simulink library "LU_TEG"  (R2015a)
settings: Solver=ode45  StartTime=0.0  StopTime=10.0  RelTol=1e-3
undefined symbols (not defined in the file): a, a_hxr, B, b_hxr, C_ap, C_cxr, C_hxr, ca1, ca2, ca3, cb1, cb2, cb3, ct1, ct2, Di_cxr, f, k_gap, l, l_cw, l_hxr, l_TEM, M, M_ap, M_cxr, M_hxr, n, N, Nf_hxr, P, plate_fin_hxr_A, side, T1, T1_T2, T_cint, T_hint, tf_hxr, Tune_er, Tune_tr
(part 1 of 2)
settings Model: Creator=lansong7  LastModifiedBy=lansong7

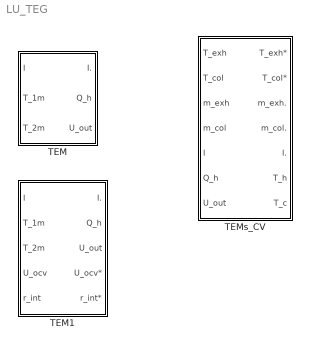
== system LU_TEG ==
  TEM : Subsystem  mask{l=l, l_cw=l_cw, f=f, a=a, n=n, Tune_tr=Tune_tr, Tune_er=Tune_er, ct1=ct1, ct2=ct2}
      mask prompts: l "Length of thermocouples [m]"; l_cw "Cermaic wafer length [m]"; f "Fill factor [-]"; a "Area of a TEM [m2]"; n "Number of thermal couple"; Tune_tr "Tuning for thermal resistance"; Tune_er "Tuning for electrical resistance"; ct1 "Tuning for  contact resistance ct1"; ct2 "Tuning for  contact resistance ct2"
      mask DialogControl ParameterGroupVar_copy Prompt: Geometrical Parameters
      mask DialogControl ParameterGroupVar Prompt: Tuning Parameters
  TEM1 : Subsystem  mask{l=l, l_cw=l_cw, f=f, a=a, n=n, Tune_tr=Tune_tr, Tune_er=Tune_er, ct1=ct1, ct2=ct2, M=M}
      mask prompts: l "Length of thermocouples [m]"; l_cw "Cermaic wafer length [m]"; f "Fill factor [-]"; a "Area of a TEM [m2]"; n "Number of thermal couple"; Tune_tr "Tuning for thermal resistance"; Tune_er "Tuning for electrical resistance"; ct1 "Tuning for  contact resistance ct1"; ct2 "Tuning for  contact resistance ct2"; M "Number of TEMs in a CV"
      mask DialogControl ParameterGroupVar_copy Prompt: Geometrical Parameters
      mask DialogControl ParameterGroupVar Prompt: Tuning Parameters
  TEMs_CV : Subsystem  mask{B=B, a=a, side=side, l_TEM=l_TEM, M=M, M_hxr=M_hxr, M_ap=M_ap, C_hxr=C_hxr, C_ap=C_ap, l_hxr=l_hxr, b_hxr=b_hxr, a_hxr=a_hxr, Nf_hxr=Nf_hxr, tf_hxr=tf_hxr, M_cxr=M_cxr, C_cxr=C_cxr, Di_cxr=Di_cxr, T_hint=T_hint, T_cint=T_cint, ca1=ca1, ca2=ca2, ca3=ca3, cb1=cb1, cb2=cb2, cb3=cb3}
      mask prompts: B "Area of a Control Volume [m2]"; a "Areas of a TEM [m2]"; side "Number of heat exchanger channels"; l_TEM "Length of  a TEM [m]"; M "Number of TEMs in a CV"; M_hxr "Mass of hot side  heat exchanger [kg]"; M_ap "Mass of aluminate plate [kg]"; C_hxr "Heat capacity of of hot side heat exchanger [J/(kg.K)]"; C_ap "Heat capacity of of aluminate plate [J/(kg.K)]"; l_hxr "Length of hot side heat exchanger [m]"; b_hxr "Width of hot side heat exchanger"; a_hxr "Height of hot side heat exchanger"; Nf_hxr "Number of the fins of hot side heat exchanger"; tf_hxr "Fin thickness of hot side heat exchanger"; M_cxr "Mass of cold side  heat exchanger [kg]"; C_cxr "Heat capacity of of cold side heat exchanger [J/(kg.K)]"; Di_cxr "Inner diameter of cold side heat exchanger"; T_hint "Initial temperature of hot side wall"; T_cint "Initial temperature of cold side wall"; ca1 "Tuning constant of hot side transfer coefficient ca1"; ca2 "Tuning constant of hot side transfer coefficient ca2"; ca3 "Tuning constant of hot side transfer coefficient ca3"; cb1 "Tuning constant of cold side transfer coefficient cb1"; cb2 "Tuning constant of cold side transfer coefficient cb2"; cb3 "Tuning constant of cold side transfer coefficient cb3"
      mask DialogControl ParameterGroupVar Prompt: Geometrical Parameters
      mask DialogControl ParameterGroupVar_copy Prompt: Hot side Heat Exchanger Parameters
      mask DialogControl ParameterGroupVar_copy_copy Prompt: Cold side Heat Exchanger Parameters
      mask DialogControl ParameterGroupVar_copy_copy_copy Prompt: Tuning Parameters

== system LU_TEG/TEM ==
  note: 2
  I : Inport  OutDataTypeStr=double  PortDimensions=1  SampleTime=[0,1]
  T_1m : Inport  Port=2  OutDataTypeStr=double  PortDimensions=1  SampleTime=[0,1]
  T_2m : Inport  Port=3  OutDataTypeStr=double  PortDimensions=1  SampleTime=[0,1]
  Spn : Subsystem
  Subsystem4 : Subsystem
  Subsystem5 : Subsystem
  Terminator : Terminator
  Terminator1 : Terminator
  r_int : Subsystem
  I. : Outport  OutDataTypeStr=double  PortDimensions=1  SampleTime=[0,1]
  Q_h : Outport  Port=2  OutDataTypeStr=double  PortDimensions=1  SampleTime=[0,1]
  U_out : Outport  Port=3
  wires:
  Subsystem4/2(Q_h) -> Q_h/1
  I/1 -> Subsystem4/6(I)
  Subsystem4/3(U_out) -> U_out/1
  Spn/1(Spn) -> Subsystem4/7(Spn)
  r_int/1(r_int) -> Subsystem4/8(r_int)
  T_2m/1 -> r_int/2(T_2m), Spn/2(T_2m), Subsystem5/2(T_2m), Subsystem4/2(T_2m)
  Subsystem5/1(Rcw1) -> Subsystem4/3(Rh)
  Subsystem5/3(Rt) -> Subsystem4/5(Rt)
  Subsystem5/2(Rcw2) -> Subsystem4/4(Rc)
  Subsystem4/4(U_ocv) -> Terminator/1
  Subsystem4/1(I.) -> I./1
  Subsystem4/5(r_int.) -> Terminator1/1
  T_1m/1 -> r_int/1(T_1m), Spn/1(T_1m), Subsystem5/1(T_1m), Subsystem4/1(T_1m)

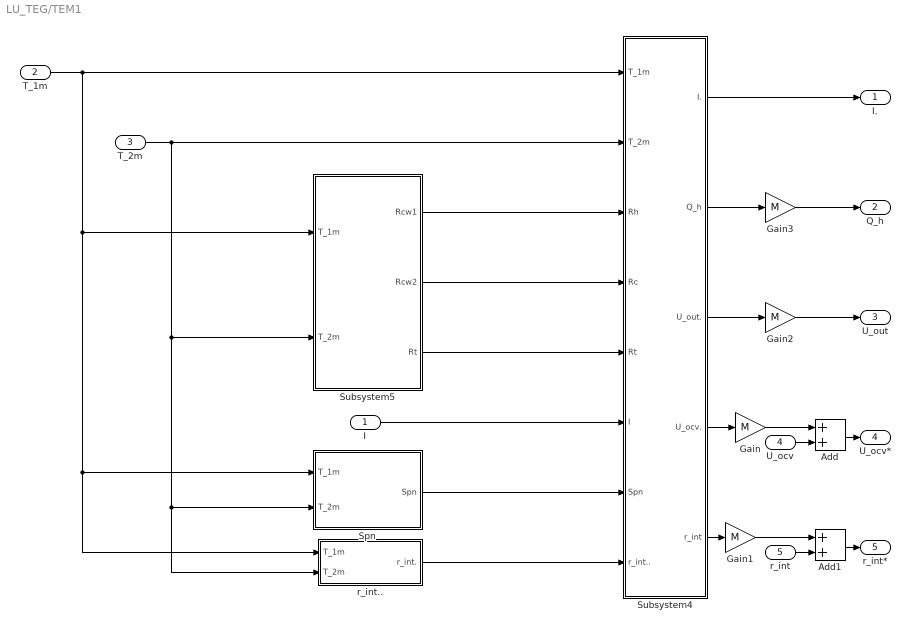
== system LU_TEG/TEM1 ==
  I : Inport  OutDataTypeStr=double  PortDimensions=1  SampleTime=[0,1]
  T_1m : Inport  Port=2  OutDataTypeStr=double  PortDimensions=1  SampleTime=[0,1]
  T_2m : Inport  Port=3  OutDataTypeStr=double  PortDimensions=1  SampleTime=[0,1]
  U_ocv : Inport  Port=4  OutDataTypeStr=double  PortDimensions=1  SampleTime=[0,1]
  r_int : Inport  Port=5  OutDataTypeStr=double  PortDimensions=1  SampleTime=[0,1]
  Add : Sum
  Add1 : Sum
  Gain{,1..3} (4 alike) : Gain  Gain=M
  Spn : Subsystem
  Subsystem4 : Subsystem
  Subsystem5 : Subsystem
  r_int.. : Subsystem
  I. : Outport  OutDataTypeStr=double  PortDimensions=1  SampleTime=[0,1]
  Q_h : Outport  Port=2  OutDataTypeStr=double  PortDimensions=1  SampleTime=[0,1]
  U_out : Outport  Port=3
  U_ocv* : Outport  Port=4
  "r_int* " : Outport  Port=5
  wires:
  T_1m/1 -> Subsystem4/1(T_1m), Subsystem5/1(T_1m), Spn/1(T_1m), r_int../1(T_1m)
  Subsystem4/1(I.) -> I./1
  Subsystem5/2(Rcw2) -> Subsystem4/4(Rc)
  Subsystem5/3(Rt) -> Subsystem4/5(Rt)
  Subsystem5/1(Rcw1) -> Subsystem4/3(Rh)
  T_2m/1 -> Subsystem4/2(T_2m), Subsystem5/2(T_2m), Spn/2(T_2m), r_int../2(T_2m)
  r_int../1(r_int.) -> Subsystem4/8(r_int..)
  Spn/1(Spn) -> Subsystem4/7(Spn)
  Subsystem4/3(U_out.) -> Gain2/1
  I/1 -> Subsystem4/6(I)
  Subsystem4/2(Q_h) -> Gain3/1
  Subsystem4/4(U_ocv.) -> Gain/1
  U_ocv/1 -> Add/2
  Subsystem4/5(r_int) -> Gain1/1
  r_int/1 -> Add1/2
  Gain2/1 -> U_out/1
  Gain3/1 -> Q_h/1
  Gain/1 -> Add/1
  Add/1 -> U_ocv*/1
  Gain1/1 -> Add1/1
  Add1/1 -> "r_int* "/1

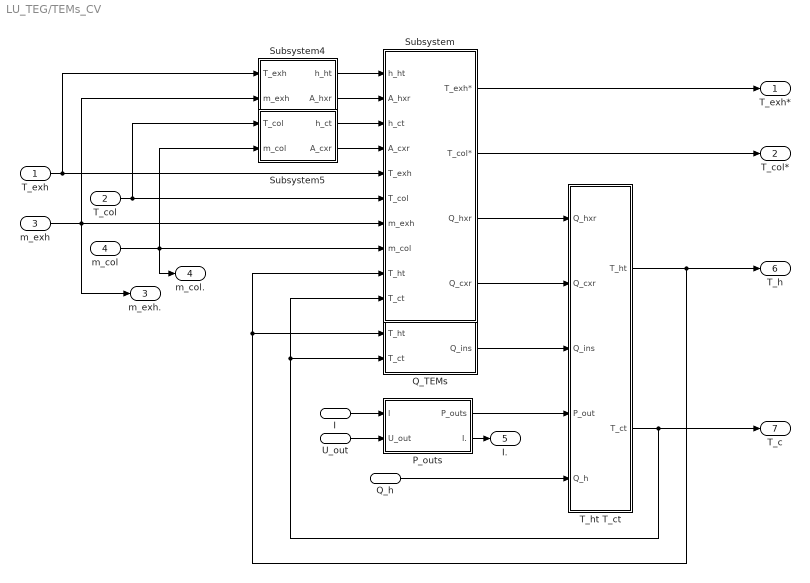
== system LU_TEG/TEMs_CV ==
  T_exh : Inport
  T_col : Inport  Port=2
  m_exh : Inport  Port=3
  m_col : Inport  Port=4
  I : Inport  Port=5
  Q_h : Inport  Port=6
  U_out : Inport  Port=7
  P_outs : Subsystem
  Q_TEMs : Subsystem
  Subsystem : Subsystem
  Subsystem4 : Subsystem
  Subsystem5 : Subsystem
  T_ht T_ct : Subsystem
  T_exh* : Outport
  T_col* : Outport  Port=2
  m_exh. : Outport  Port=3
  m_col. : Outport  Port=4
  I. : Outport  Port=5
  T_h : Outport  Port=6
  T_c : Outport  Port=7
  wires:
  T_exh/1 -> Subsystem4/1(T_exh), Subsystem/5(T_exh)
  T_col/1 -> Subsystem5/1(T_col), Subsystem/6(T_col)
  m_exh/1 -> Subsystem4/2(m_exh), Subsystem/7(m_exh), m_exh./1
  m_col/1 -> m_col./1, Subsystem5/2(m_col), Subsystem/8(m_col)
  Subsystem/1(T_exh*) -> T_exh*/1
  Subsystem/2(T_col*) -> T_col*/1
  Q_TEMs/1(Q_ins) -> T_ht T_ct/3(Q_ins)
  Subsystem/3(Q_hxr) -> T_ht T_ct/1(Q_hxr)
  Subsystem/4(Q_cxr) -> T_ht T_ct/2(Q_cxr)
  I/1 -> P_outs/1(I)
  U_out/1 -> P_outs/2(U_out)
  P_outs/1(P_outs) -> T_ht T_ct/4(P_out)
  P_outs/2(I.) -> I./1
  T_ht T_ct/2(T_ct) -> Subsystem/10(T_ct), Q_TEMs/2(T_ct), T_c/1
  T_ht T_ct/1(T_ht) -> Subsystem/9(T_ht), Q_TEMs/1(T_ht), T_h/1
  Subsystem4/2(A_hxr) -> Subsystem/2(A_hxr)
  Subsystem5/1(h_ct) -> Subsystem/3(h_ct)
  Subsystem5/2(A_cxr) -> Subsystem/4(A_cxr)
  Subsystem4/1(h_ht) -> Subsystem/1(h_ht)
  Q_h/1 -> T_ht T_ct/5(Q_h)

== system LU_TEG/TEM/Spn ==
  T_1m : Inport
  T_2m : Inport  Port=2
  Add : Sum  Inputs=+-
  Add2 : Sum
  Constant2 : Constant  Value=n
  Gain : Gain  Gain=0.5
  Product : Product
  sn : Lookup_n-D  NumberOfTableDimensions=1  BreakpointsForDimension1=N(:,1)  Table=N(:,2)  InterpMethod=Cubic spline  ExtrapMethod=Cubic spline  InternalRulePriority=Speed  RndMeth=Simplest  InputSameDT=on
  sp : Lookup_n-D  NumberOfTableDimensions=1  BreakpointsForDimension1=P(:,1)  Table=P(:,2)  InterpMethod=Cubic spline  ExtrapMethod=Cubic spline  InternalRulePriority=Speed  RndMeth=Simplest  InputSameDT=on
  Spn : Outport
  wires:
  sn/1 -> Add/2
  sp/1 -> Add/1
  Constant2/1 -> Product/1
  Product/1 -> Spn/1
  Add2/1 -> Gain/1
  Gain/1 -> sp/1, sn/1
  T_1m/1 -> Add2/1
  T_2m/1 -> Add2/2
  Add/1 -> Product/2

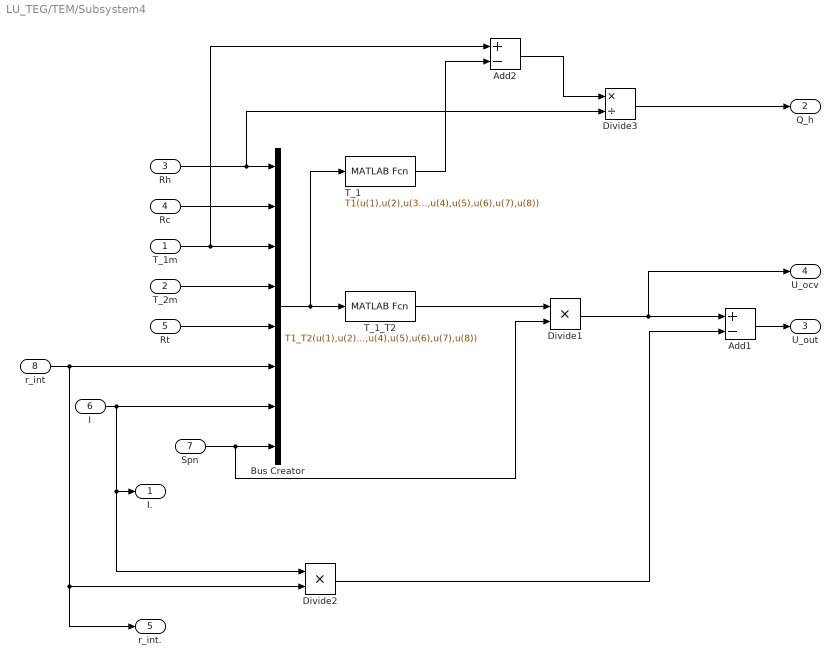
== system LU_TEG/TEM/Subsystem4 ==
  T_1m : Inport
  T_2m : Inport  Port=2
  Rh : Inport  Port=3
  Rc : Inport  Port=4
  Rt : Inport  Port=5
  I : Inport  Port=6
  Spn : Inport  Port=7
  r_int : Inport  Port=8
  Add1 : Sum  Inputs=+-
  Add2 : Sum  Inputs=+-
  Bus Creator : BusCreator  Inputs=8
  Divide1 : Product  Inputs=**
  Divide2 : Product  Inputs=**
  Divide3 : Product  Inputs=*/
  T_1 : MATLABFcn  MATLABFcn=T1(u(1),u(2),u(3),u(4),u(5),u(6),u(7),u(8))  OutputSignalType=real
  T_1_T2 : MATLABFcn  MATLABFcn=T1_T2(u(1),u(2),u(3),u(4),u(5),u(6),u(7),u(8))  OutputSignalType=real
  I. : Outport  OutDataTypeStr=double  PortDimensions=1  SampleTime=[0,1]
  Q_h : Outport  Port=2  OutDataTypeStr=double  PortDimensions=1  SampleTime=[0,1]
  U_out : Outport  Port=3
  U_ocv : Outport  Port=4
  r_int. : Outport  Port=5  OutDataTypeStr=double  PortDimensions=1  SampleTime=[0,1]
  wires:
  r_int/1 -> Bus Creator/6, Divide2/2, r_int./1
  Rh/1 -> Divide3/2, Bus Creator/1
  Rc/1 -> Bus Creator/2
  Rt/1 -> Bus Creator/5
  T_2m/1 -> Bus Creator/4
  T_1m/1 -> Add2/1, Bus Creator/3
  I/1 -> Bus Creator/7, Divide2/1, I./1
  Divide2/1 -> Add1/2
  Add1/1 -> U_out/1
  Spn/1 -> Bus Creator/8, Divide1/2
  Divide1/1 -> U_ocv/1, Add1/1
  T_1_T2/1 -> Divide1/1
  Bus Creator/1 -> T_1/1, T_1_T2/1
  T_1/1 -> Add2/2
  Divide3/1 -> Q_h/1
  Add2/1 -> Divide3/1

== system LU_TEG/TEM/Subsystem5 ==
  T_1m : Inport
  T_2m : Inport  Port=2
  R_cw : Subsystem
  Rt. : Subsystem
  Rcw1 : Outport
  Rcw2 : Outport  Port=2
  Rt : Outport  Port=3
  wires:
  R_cw/1(Rcw1) -> Rcw1/1
  Rt./1(Rt) -> Rt/1
  R_cw/2(Rcw2) -> Rcw2/1
  T_2m/1 -> R_cw/2(T_2m), Rt./2(T_2m)
  T_1m/1 -> R_cw/1(T_1m), Rt./1(T_1m)

== system LU_TEG/TEM/r_int ==
  T_1m : Inport
  T_2m : Inport  Port=2
  Add2 : Sum
  Add4 : Sum
  Constant12 : Constant  Value=0.5*a*f/n
  Constant13 : Constant  Value=0.5*a*f/n
  Constant14 : Constant  Value=l
  Constant16 : Constant  Value=l
  Constant18 : Constant  Value=n
  Constant4 : Constant  Value=n
  Gain : Gain  Gain=Tune_er
  Gain1 : Gain  Gain=0.5
  Product3 : Product  Inputs=***/
  Product4 : Product  Inputs=***/
  rhon : Lookup_n-D  NumberOfTableDimensions=1  BreakpointsForDimension1=N(:,1)  Table=N(:,3)  InterpMethod=Cubic spline  ExtrapMethod=Cubic spline  InternalRulePriority=Speed  RndMeth=Simplest  InputSameDT=on
  rhop : Lookup_n-D  NumberOfTableDimensions=1  BreakpointsForDimension1=P(:,1)  Table=P(:,3)  InterpMethod=Cubic spline  ExtrapMethod=Cubic spline  InternalRulePriority=Speed  RndMeth=Simplest  InputSameDT=on
  r_int : Outport
  wires:
  Constant18/1 -> Product4/1
  Constant14/1 -> Product3/2
  rhop/1 -> Product3/3
  Constant12/1 -> Product3/4
  rhon/1 -> Product4/3
  Constant13/1 -> Product4/4
  Constant4/1 -> Product3/1
  Constant16/1 -> Product4/2
  Product3/1 -> Add2/1
  Product4/1 -> Add2/2
  T_1m/1 -> Add4/1
  T_2m/1 -> Add4/2
  Add4/1 -> Gain1/1
  Add2/1 -> Gain/1
  Gain1/1 -> rhon/1, rhop/1
  Gain/1 -> r_int/1

== system LU_TEG/TEM1/Spn ==
  T_1m : Inport
  T_2m : Inport  Port=2
  Add : Sum  Inputs=+-
  Add2 : Sum
  Constant2 : Constant  Value=n
  Gain : Gain  Gain=0.5
  Product : Product
  sn : Lookup_n-D  NumberOfTableDimensions=1  BreakpointsForDimension1=N(:,1)  Table=N(:,2)  InterpMethod=Cubic spline  ExtrapMethod=Cubic spline  InternalRulePriority=Speed  RndMeth=Simplest  InputSameDT=on
  sp : Lookup_n-D  NumberOfTableDimensions=1  BreakpointsForDimension1=P(:,1)  Table=P(:,2)  InterpMethod=Cubic spline  ExtrapMethod=Cubic spline  InternalRulePriority=Speed  RndMeth=Simplest  InputSameDT=on
  Spn : Outport
  wires:
  Add/1 -> Product/2
  T_2m/1 -> Add2/2
  T_1m/1 -> Add2/1
  Gain/1 -> sn/1, sp/1
  Add2/1 -> Gain/1
  Product/1 -> Spn/1
  Constant2/1 -> Product/1
  sp/1 -> Add/1
  sn/1 -> Add/2

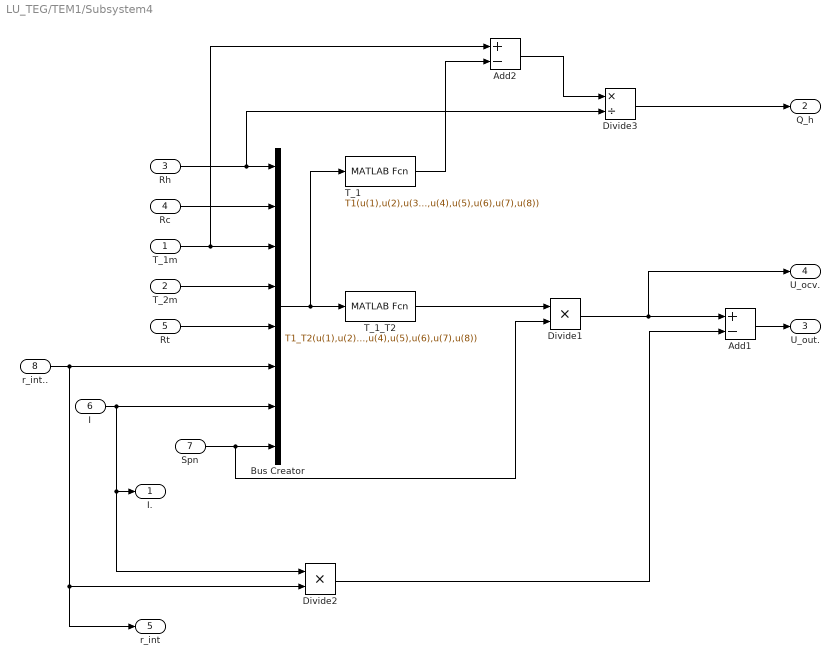
== system LU_TEG/TEM1/Subsystem4 ==
  T_1m : Inport
  T_2m : Inport  Port=2
  Rh : Inport  Port=3
  Rc : Inport  Port=4
  Rt : Inport  Port=5
  I : Inport  Port=6
  Spn : Inport  Port=7
  r_int.. : Inport  Port=8
  Add1 : Sum  Inputs=+-
  Add2 : Sum  Inputs=+-
  Bus Creator : BusCreator  Inputs=8
  Divide1 : Product  Inputs=**
  Divide2 : Product  Inputs=**
  Divide3 : Product  Inputs=*/
  T_1 : MATLABFcn  MATLABFcn=T1(u(1),u(2),u(3),u(4),u(5),u(6),u(7),u(8))  OutputSignalType=real
  T_1_T2 : MATLABFcn  MATLABFcn=T1_T2(u(1),u(2),u(3),u(4),u(5),u(6),u(7),u(8))  OutputSignalType=real
  I. : Outport  OutDataTypeStr=double  PortDimensions=1  SampleTime=[0,1]
  Q_h : Outport  Port=2  OutDataTypeStr=double  PortDimensions=1  SampleTime=[0,1]
  U_out. : Outport  Port=3
  U_ocv. : Outport  Port=4
  r_int : Outport  Port=5  OutDataTypeStr=double  PortDimensions=1  SampleTime=[0,1]
  wires:
  Add2/1 -> Divide3/1
  Divide3/1 -> Q_h/1
  T_1/1 -> Add2/2
  Bus Creator/1 -> T_1_T2/1, T_1/1
  T_1_T2/1 -> Divide1/1
  Divide1/1 -> Add1/1, U_ocv./1
  Spn/1 -> Divide1/2, Bus Creator/8
  Add1/1 -> U_out./1
  Divide2/1 -> Add1/2
  I/1 -> I./1, Divide2/1, Bus Creator/7
  T_1m/1 -> Bus Creator/3, Add2/1
  T_2m/1 -> Bus Creator/4
  Rt/1 -> Bus Creator/5
  Rc/1 -> Bus Creator/2
  Rh/1 -> Bus Creator/1, Divide3/2
  r_int../1 -> r_int/1, Divide2/2, Bus Creator/6

== system LU_TEG/TEM1/Subsystem5 ==
  T_1m : Inport
  T_2m : Inport  Port=2
  R_cw : Subsystem
  Rt. : Subsystem
  Rcw1 : Outport
  Rcw2 : Outport  Port=2
  Rt : Outport  Port=3
  wires:
  T_1m/1 -> Rt./1(T_1m), R_cw/1(T_1m)
  T_2m/1 -> Rt./2(T_2m), R_cw/2(T_2m)
  R_cw/2(Rcw2) -> Rcw2/1
  Rt./1(Rt) -> Rt/1
  R_cw/1(Rcw1) -> Rcw1/1

== system LU_TEG/TEM1/r_int.. ==
  T_1m : Inport
  T_2m : Inport  Port=2
  Add2 : Sum
  Add4 : Sum
  Constant12 : Constant  Value=0.5*a*f/n
  Constant13 : Constant  Value=0.5*a*f/n
  Constant14 : Constant  Value=l
  Constant16 : Constant  Value=l
  Constant18 : Constant  Value=n
  Constant4 : Constant  Value=n
  Gain : Gain  Gain=Tune_er
  Gain1 : Gain  Gain=0.5
  Product3 : Product  Inputs=***/
  Product4 : Product  Inputs=***/
  rhon : Lookup_n-D  NumberOfTableDimensions=1  BreakpointsForDimension1=N(:,1)  Table=N(:,3)  InterpMethod=Cubic spline  ExtrapMethod=Cubic spline  InternalRulePriority=Speed  RndMeth=Simplest  InputSameDT=on
  rhop : Lookup_n-D  NumberOfTableDimensions=1  BreakpointsForDimension1=P(:,1)  Table=P(:,3)  InterpMethod=Cubic spline  ExtrapMethod=Cubic spline  InternalRulePriority=Speed  RndMeth=Simplest  InputSameDT=on
  r_int. : Outport
  wires:
  Gain/1 -> r_int./1
  Gain1/1 -> rhop/1, rhon/1
  Add2/1 -> Gain/1
  Add4/1 -> Gain1/1
  T_2m/1 -> Add4/2
  T_1m/1 -> Add4/1
  Product4/1 -> Add2/2
  Product3/1 -> Add2/1
  Constant16/1 -> Product4/2
  Constant4/1 -> Product3/1
  Constant13/1 -> Product4/4
  rhon/1 -> Product4/3
  Constant12/1 -> Product3/4
  rhop/1 -> Product3/3
  Constant14/1 -> Product3/2
  Constant18/1 -> Product4/1

== system LU_TEG/TEMs_CV/P_outs ==
  I : Inport
  U_out : Inport  Port=2
  Divide : Product  Inputs=**
  P_outs : Outport
  I. : Outport  Port=2
  wires:
  Divide/1 -> P_outs/1
  I/1 -> I./1, Divide/2
  U_out/1 -> Divide/1

== system LU_TEG/TEMs_CV/Q_TEMs ==
  T_ht : Inport
  T_ct : Inport  Port=2
  Q_TEMs. : Subsystem
  Q_ins : Outport
  wires:
  T_ht/1 -> Q_TEMs./1(T_ht)
  T_ct/1 -> Q_TEMs./2(T_ct)
  Q_TEMs./1(Q_ins) -> Q_ins/1

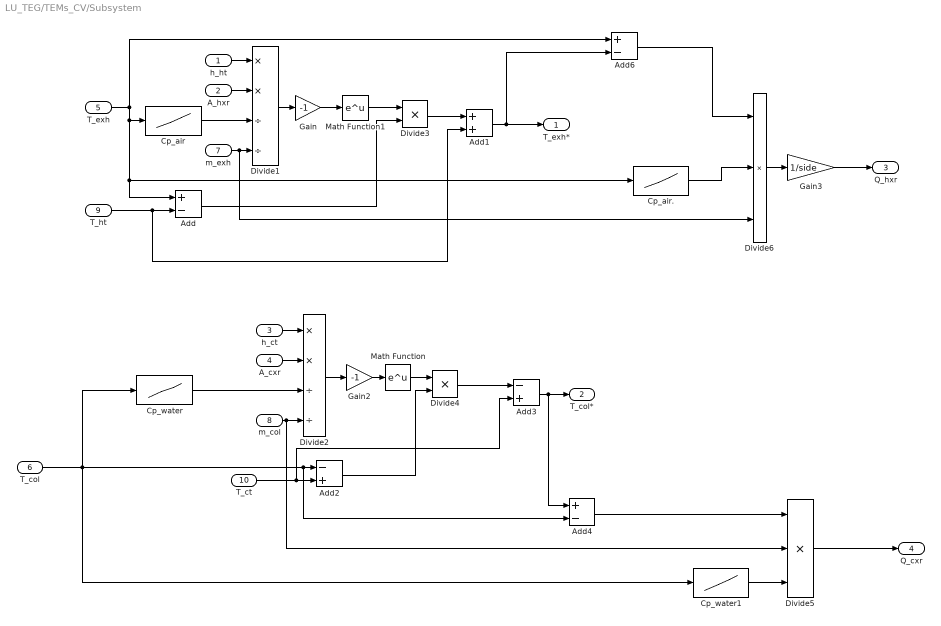
== system LU_TEG/TEMs_CV/Subsystem ==
  h_ht : Inport
  A_hxr : Inport  Port=2
  h_ct : Inport  Port=3
  A_cxr : Inport  Port=4
  T_exh : Inport  Port=5
  T_col : Inport  Port=6
  m_exh : Inport  Port=7
  m_col : Inport  Port=8
  T_ht : Inport  Port=9
  T_ct : Inport  Port=10
  Add : Sum  Inputs=+-
  Add1 : Sum
  Add2 : Sum  Inputs=-+
  Add3 : Sum  Inputs=-+
  Add4 : Sum  Inputs=+-
  Add6 : Sum  Inputs=+-
  Cp_air : Lookup_n-D  NumberOfTableDimensions=1  BreakpointsForDimension1=|  Table=|  InterpMethod=Cubic spline  ExtrapMethod=Cubic spline  RndMeth=Simplest  InputSameDT=on
      BreakpointsForDimension1=|
      | [293
      | 313
      | 333
      | 353
      | 373
      | 393
      | 413
      | 433
      | 453
      | 473
      | 493
      | 513
      | 533
      | 553
      | 573
      | 593
      | 613
      | 633
      | 653
      | 673
      | 693
      | 713
      | 733
      | 753
      | 773
      | 793
      | 813
      | 833
      | 853
      | 873
      | 900
      | 920
      | 940
      | 960
      | 980
      | 1000
      | 1020
      | 1040
      | 1060
      | 1080
      | 1100
      | 1120
      | 1140
      | 1160
      | 1180
      | 1200
      | 1220
      | 1240
      | 1260
      | 1280
      | 1300
      | 1320
      | 1340
      | 1360
      | 1380
      | 1400
      | 1420
      | 1440
      | 1460
      | 1480]
      Table=|
      | [1007
      | 1008
      | 1008
      | 1009
      | 1011
      | 1013
      | 1016
      | 1019
      | 1023
      | 1026
      | 1029
      | 1033
      | 1036
      | 1041
      | 1046
      | 1050
      | 1055
      | 1059
      | 1064
      | 1069
      | 1073
      | 1078
      | 1082
      | 1088
      | 1093
      | 1097
      | 1102
      | 1106
      | 1111
      | 1115
      | 1121
      | 1125
      | 1129
      | 1133
      | 1137
      | 1141
      | 1145
      | 1148
      | 1152
      | 1155
      | 1159
      | 1162
      | 1165
      | 1168
      | 1171
      | 1174
      | 1177
      | 1180
      | 1183
      | 1185
      | 1188
      | 1191
      | 1193
      | 1196
      | 1198
      | 1200
      | 1202
      | 1205
      | 1207
      | 1209
      | ]
  Cp_air. : Lookup_n-D  NumberOfTableDimensions=1  BreakpointsForDimension1=|  Table=|  InterpMethod=Cubic spline  ExtrapMethod=Cubic spline  RndMeth=Simplest  InputSameDT=on
      BreakpointsForDimension1=|
      | [293
      | 313
      | 333
      | 353
      | 373
      | 393
      | 413
      | 433
      | 453
      | 473
      | 493
      | 513
      | 533
      | 553
      | 573
      | 593
      | 613
      | 633
      | 653
      | 673
      | 693
      | 713
      | 733
      | 753
      | 773
      | 793
      | 813
      | 833
      | 853
      | 873
      | 900
      | 920
      | 940
      | 960
      | 980
      | 1000
      | 1020
      | 1040
      | 1060
      | 1080
      | 1100
      | 1120
      | 1140
      | 1160
      | 1180
      | 1200
      | 1220
      | 1240
      | 1260
      | 1280
      | 1300
      | 1320
      | 1340
      | 1360
      | 1380
      | 1400
      | 1420
      | 1440
      | 1460
      | 1480]
      Table=|
      | [1007
      | 1008
      | 1008
      | 1009
      | 1011
      | 1013
      | 1016
      | 1019
      | 1023
      | 1026
      | 1029
      | 1033
      | 1036
      | 1041
      | 1046
      | 1050
      | 1055
      | 1059
      | 1064
      | 1069
      | 1073
      | 1078
      | 1082
      | 1088
      | 1093
      | 1097
      | 1102
      | 1106
      | 1111
      | 1115
      | 1121
      | 1125
      | 1129
      | 1133
      | 1137
      | 1141
      | 1145
      | 1148
      | 1152
      | 1155
      | 1159
      | 1162
      | 1165
      | 1168
      | 1171
      | 1174
      | 1177
      | 1180
      | 1183
      | 1185
      | 1188
      | 1191
      | 1193
      | 1196
      | 1198
      | 1200
      | 1202
      | 1205
      | 1207
      | 1209
      | ]
  Cp_water : Lookup_n-D  NumberOfTableDimensions=1  BreakpointsForDimension1=|  Table=|  InterpMethod=Cubic spline  ExtrapMethod=Cubic spline  RndMeth=Simplest  InputSameDT=on
      BreakpointsForDimension1=|
      | [273
      | 274
      | 275
      | 276
      | 277
      | 278
      | 279
      | 280
      | 281
      | 282
      | 283
      | 284
      | 285
      | 286
      | 287
      | 288
      | 289
      | 290
      | 291
      | 292
      | 293
      | 294
      | 295
      | 296
      | 297
      | 298
      | 299
      | 300
      | 301
      | 302
      | 303
      | 304
      | 305
      | 306
      | 307
      | 308
      | 309
      | 310
      | 311
      | 312
      | 313
      | 314
      | 315
      | 316
      | 317
      | 318
      | 319
      | 320
      | 321
      | 322
      | 323
      | 324
      | 325
      | 326
      | 327
      | 328
      | 329
      | 330
      | 331
      | 332
      | 333
      | 334
      | 335
      | 336
      | 337
      | 338
      | 339
      | 340
      | 341
      | 342
      | 343
      | 344
      | 345
      | 346
      | 347
      | 348
      | 349
      | 350
      | 351
      | 352
      | 353
      | 354
      | 355
      | 356
      | 357
      | 358
      | 359
      | 360
      | 361
      | 362
      | 363
      | 364
      | 365
      | 366
      | 367
      | 368
      | 369
      | 370
      | 371
      | 372
      | 373]
      Table=|
      | [4217
      | 4213
      | 4210
      | 4207
      | 4205
      | 4202
      | 4200
      | 4198
      | 4196
      | 4194
      | 4192
      | 4191
      | 4189
      | 4188
      | 4187
      | 4186
      | 4185
      | 4184
      | 4183
      | 4182
      | 4182
      | 4181
      | 4181
      | 4180
      | 4180
      | 4180
      | 4179
      | 4179
      | 4179
      | 4179
      | 4178
      | 4178
      | 4178
      | 4178
      | 4178
      | 4178
      | 4178
      | 4178
      | 4178
      | 4179
      | 4179
      | 4179
      | 4179
      | 4179
      | 4179
      | 4180
      | 4180
      | 4180
      | 4180
      | 4181
      | 4181
      | 4181
      | 4182
      | 4182
      | 4182
      | 4183
      | 4183
      | 4183
      | 4184
      | 4184
      | 4185
      | 4185
      | 4186
      | 4186
      | 4187
      | 4187
      | 4188
      | 4188
      | 4189
      | 4189
      | 4190
      | 4190
      | 4191
      | 4192
      | 4192
      | 4193
      | 4194
      | 4194
      | 4195
      | 4196
      | 4196
      | 4197
      | 4198
      | 4199
      | 4200
      | 4200
      | 4201
      | 4202
      | 4203
      | 4204
      | 4205
      | 4206
      | 4207
      | 4208
      | 4209
      | 4210
      | 4211
      | 4212
      | 4213
      | 4214
      | 4216]
  Cp_water1 : Lookup_n-D  NumberOfTableDimensions=1  BreakpointsForDimension1=|  Table=|  InterpMethod=Cubic spline  ExtrapMethod=Cubic spline  RndMeth=Simplest  InputSameDT=on
      BreakpointsForDimension1=|
      | [273
      | 274
      | 275
      | 276
      | 277
      | 278
      | 279
      | 280
      | 281
      | 282
      | 283
      | 284
      | 285
      | 286
      | 287
      | 288
      | 289
      | 290
      | 291
      | 292
      | 293
      | 294
      | 295
      | 296
      | 297
      | 298
      | 299
      | 300
      | 301
      | 302
      | 303
      | 304
      | 305
      | 306
      | 307
      | 308
      | 309
      | 310
      | 311
      | 312
      | 313
      | 314
      | 315
      | 316
      | 317
      | 318
      | 319
      | 320
      | 321
      | 322
      | 323
      | 324
      | 325
      | 326
      | 327
      | 328
      | 329
      | 330
      | 331
      | 332
      | 333
      | 334
      | 335
      | 336
      | 337
      | 338
      | 339
      | 340
      | 341
      | 342
      | 343
      | 344
      | 345
      | 346
      | 347
      | 348
      | 349
      | 350
      | 351
      | 352
      | 353
      | 354
      | 355
      | 356
      | 357
      | 358
      | 359
      | 360
      | 361
      | 362
      | 363
      | 364
      | 365
      | 366
      | 367
      | 368
      | 369
      | 370
      | 371
      | 372
      | 373]
      Table=|
      | [4217
      | 4213
      | 4210
      | 4207
      | 4205
      | 4202
      | 4200
      | 4198
      | 4196
      | 4194
      | 4192
      | 4191
      | 4189
      | 4188
      | 4187
      | 4186
      | 4185
      | 4184
      | 4183
      | 4182
      | 4182
      | 4181
      | 4181
      | 4180
      | 4180
      | 4180
      | 4179
      | 4179
      | 4179
      | 4179
      | 4178
      | 4178
      | 4178
      | 4178
      | 4178
      | 4178
      | 4178
      | 4178
      | 4178
      | 4179
      | 4179
      | 4179
      | 4179
      | 4179
      | 4179
      | 4180
      | 4180
      | 4180
      | 4180
      | 4181
      | 4181
      | 4181
      | 4182
      | 4182
      | 4182
      | 4183
      | 4183
      | 4183
      | 4184
      | 4184
      | 4185
      | 4185
      | 4186
      | 4186
      | 4187
      | 4187
      | 4188
      | 4188
      | 4189
      | 4189
      | 4190
      | 4190
      | 4191
      | 4192
      | 4192
      | 4193
      | 4194
      | 4194
      | 4195
      | 4196
      | 4196
      | 4197
      | 4198
      | 4199
      | 4200
      | 4200
      | 4201
      | 4202
      | 4203
      | 4204
      | 4205
      | 4206
      | 4207
      | 4208
      | 4209
      | 4210
      | 4211
      | 4212
      | 4213
      | 4214
      | 4216]
  Divide1 : Product  Inputs=**//
  Divide2 : Product  Inputs=**//
  Divide3 : Product  Inputs=**
  Divide4 : Product  Inputs=**
  Divide5 : Product  Inputs=***
  Divide6 : Product  Inputs=***
  Gain : Gain  Gain=-1
  Gain2 : Gain  Gain=-1
  Gain3 : Gain  Gain=1/side
  Math Function : Math  SaturateOnIntegerOverflow=on
  Math Function1 : Math  SaturateOnIntegerOverflow=on
  T_exh* : Outport
  T_col* : Outport  Port=2
  Q_hxr : Outport  Port=3
  Q_cxr : Outport  Port=4
  wires:
  Gain/1 -> Math Function1/1
  A_hxr/1 -> Divide1/2
  Add/1 -> Divide3/2
  m_col/1 -> Divide5/2, Divide2/4
  Divide4/1 -> Add3/1
  T_ht/1 -> Add1/2, Add/2
  Math Function1/1 -> Divide3/1
  Divide3/1 -> Add1/1
  Add1/1 -> Add6/2, T_exh*/1
  Add2/1 -> Divide4/2
  h_ht/1 -> Divide1/1
  Divide2/1 -> Gain2/1
  Cp_air/1 -> Divide1/3
  Add3/1 -> Add4/1, T_col*/1
  Cp_water/1 -> Divide2/3
  h_ct/1 -> Divide2/1
  A_cxr/1 -> Divide2/2
  Divide1/1 -> Gain/1
  m_exh/1 -> Divide6/3, Divide1/4
  Math Function/1 -> Divide4/1
  T_ct/1 -> Add3/2, Add2/2
  Gain2/1 -> Math Function/1
  Cp_water1/1 -> Divide5/3
  Add4/1 -> Divide5/1
  T_exh/1 -> Cp_air./1, Add/1, Cp_air/1, Add6/1
  Cp_air./1 -> Divide6/2
  Add6/1 -> Divide6/1
  Divide6/1 -> Gain3/1
  Gain3/1 -> Q_hxr/1
  Divide5/1 -> Q_cxr/1
  T_col/1 -> Cp_water1/1, Add4/2, Add2/1, Cp_water/1

== system LU_TEG/TEMs_CV/Subsystem4 ==
  T_exh : Inport
  m_exh : Inport  Port=2
  A. : MATLABFcn  MATLABFcn=plate_fin_hxr_A(u(1),u(2),u(3),u(4),u(5),u(6),u(7))
  Bus Creator1 : BusCreator  Inputs=7
  Constant2 : Constant  Value=l_hxr
  Constant3 : Constant  Value=b_hxr
  Constant4 : Constant  Value=a_hxr
  Constant5 : Constant  Value=Nf_hxr
  Constant6 : Constant  Value=tf_hxr
  Subsystem3 : Subsystem
  k_stainless : Lookup_n-D  NumberOfTableDimensions=1  BreakpointsForDimension1=|  Table=|  InterpMethod=Cubic spline  ExtrapMethod=Cubic spline  RndMeth=Simplest  InputSameDT=on
      BreakpointsForDimension1=|
      | [100.0
      | 200.0
      | 300.0
      | 400.0
      | 600.0
      | 800.0
      | 1000.0
      | 1200.0
      | 1500.0
      | ]
      Table=|
      | [9.2
      | 12.6
      | 14.9
      | 16.6
      | 19.8
      | 22.6
      | 25.4
      | 28.0
      | 31.7
      | ]
  h_ht : Outport
  A_hxr : Outport  Port=2
  wires:
  Constant6/1 -> Bus Creator1/5
  Constant2/1 -> Bus Creator1/1
  k_stainless/1 -> Bus Creator1/6
  Constant5/1 -> Bus Creator1/4
  m_exh/1 -> Subsystem3/2(m_exh)
  Constant4/1 -> Bus Creator1/3
  Bus Creator1/1 -> A./1
  Constant3/1 -> Bus Creator1/2
  A./1 -> A_hxr/1
  Subsystem3/1(h_exh) -> h_ht/1, Bus Creator1/7
  T_exh/1 -> k_stainless/1, Subsystem3/1(T_exh)

== system LU_TEG/TEMs_CV/Subsystem5 ==
  T_col : Inport
  m_col : Inport  Port=2
  Constant : Constant  Value=l_hxr*b_hxr
  Subsystem3 : Subsystem
  h_ct : Outport
  A_cxr : Outport  Port=2
  wires:
  m_col/1 -> Subsystem3/2(m_col)
  Constant/1 -> A_cxr/1
  Subsystem3/1(h_col) -> h_ct/1
  T_col/1 -> Subsystem3/1(T_col)

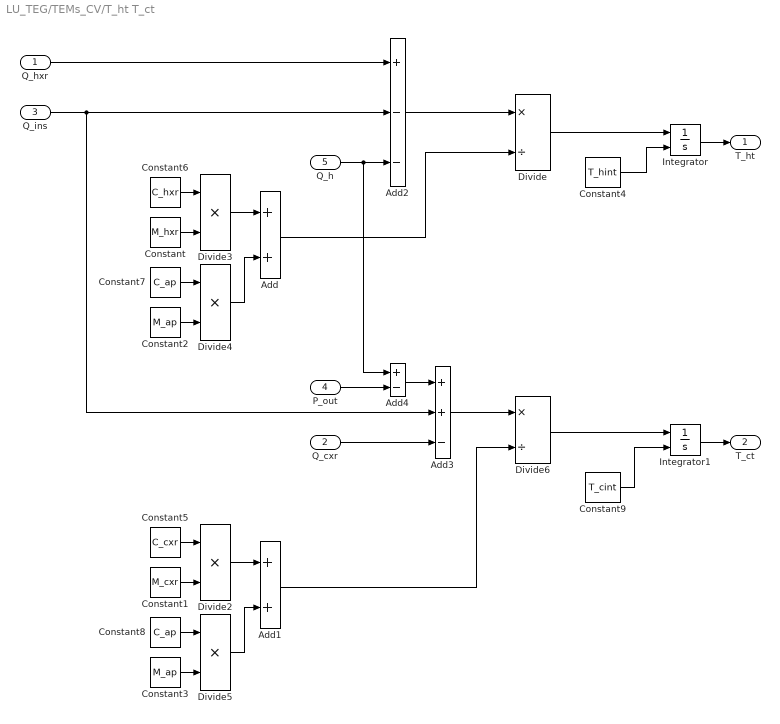
== system LU_TEG/TEMs_CV/T_ht T_ct ==
  Q_hxr : Inport
  Q_cxr : Inport  Port=2
  Q_ins : Inport  Port=3
  P_out : Inport  Port=4
  Q_h : Inport  Port=5
  Add : Sum
  Add1 : Sum
  Add2 : Sum  Inputs=+--
  Add3 : Sum  Inputs=++-
  Add4 : Sum  Inputs=+-
  Constant : Constant  Value=M_hxr
  Constant1 : Constant  Value=M_cxr
  Constant2 : Constant  Value=M_ap
  Constant3 : Constant  Value=M_ap
  Constant4 : Constant  Value=T_hint
  Constant5 : Constant  Value=C_cxr
  Constant6 : Constant  Value=C_hxr
  Constant7 : Constant  Value=C_ap
  Constant8 : Constant  Value=C_ap
  Constant9 : Constant  Value=T_cint
  Divide : Product  Inputs=*/
  Divide{2..5} (4 alike) : Product  Inputs=**
  Divide6 : Product  Inputs=*/
  Integrator : Integrator  InitialConditionSource=external
  Integrator1 : Integrator  InitialConditionSource=external
  T_ht : Outport
  T_ct : Outport  Port=2
  wires:
  Constant/1 -> Divide3/2
  Constant6/1 -> Divide3/1
  Constant7/1 -> Divide4/1
  Constant2/1 -> Divide4/2
  Divide3/1 -> Add/1
  Divide4/1 -> Add/2
  Constant1/1 -> Divide2/2
  Constant5/1 -> Divide2/1
  Constant8/1 -> Divide5/1
  Constant3/1 -> Divide5/2
  Divide2/1 -> Add1/1
  Divide5/1 -> Add1/2
  Add2/1 -> Divide/1
  Add/1 -> Divide/2
  Add3/1 -> Divide6/1
  Add1/1 -> Divide6/2
  Divide/1 -> Integrator/1
  Divide6/1 -> Integrator1/1
  Constant4/1 -> Integrator/2
  Constant9/1 -> Integrator1/2
  Integrator/1 -> T_ht/1
  Integrator1/1 -> T_ct/1
  Q_ins/1 -> Add3/2, Add2/2
  Q_hxr/1 -> Add2/1
  Q_h/1 -> Add4/1, Add2/3
  Q_cxr/1 -> Add3/3
  P_out/1 -> Add4/2
  Add4/1 -> Add3/1

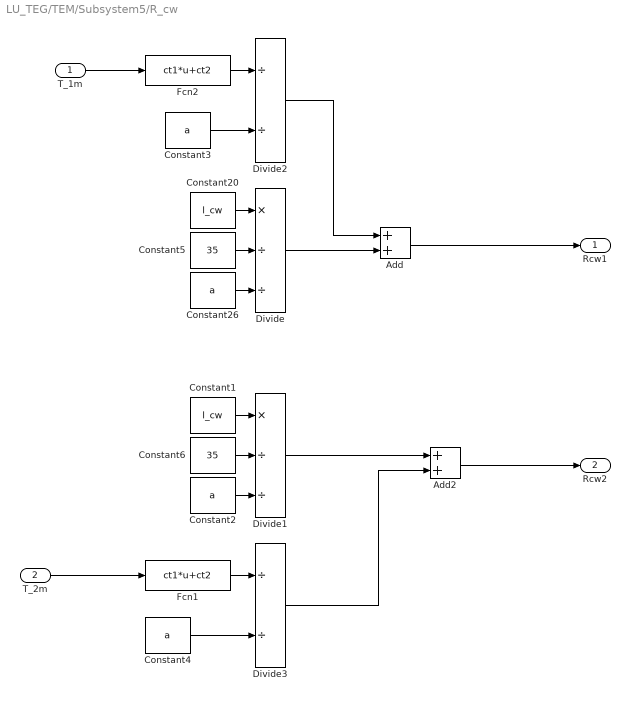
== system LU_TEG/TEM/Subsystem5/R_cw ==
  T_1m : Inport
  T_2m : Inport  Port=2
  Add : Sum
  Add2 : Sum
  Constant1 : Constant  Value=l_cw
  Constant{2..4,26} (4 alike) : Constant  Value=a
  Constant20 : Constant  Value=l_cw
  Constant5 : Constant  Value=35
  Constant6 : Constant  Value=35
  Divide : Product  Inputs=*//
  Divide1 : Product  Inputs=*//
  Divide2 : Product  Inputs=//
  Divide3 : Product  Inputs=//
  Fcn1 : Fcn  Expr=ct1*u+ct2
  Fcn2 : Fcn  Expr=ct1*u+ct2
  Rcw1 : Outport
  Rcw2 : Outport  Port=2
  wires:
  Constant20/1 -> Divide/1
  Constant26/1 -> Divide/3
  Constant5/1 -> Divide/2
  Divide/1 -> Add/2
  T_2m/1 -> Fcn1/1
  T_1m/1 -> Fcn2/1
  Constant1/1 -> Divide1/1
  Constant2/1 -> Divide1/3
  Constant6/1 -> Divide1/2
  Divide1/1 -> Add2/1
  Add/1 -> Rcw1/1
  Fcn2/1 -> Divide2/1
  Constant3/1 -> Divide2/2
  Divide2/1 -> Add/1
  Fcn1/1 -> Divide3/1
  Constant4/1 -> Divide3/2
  Divide3/1 -> Add2/2
  Add2/1 -> Rcw2/1

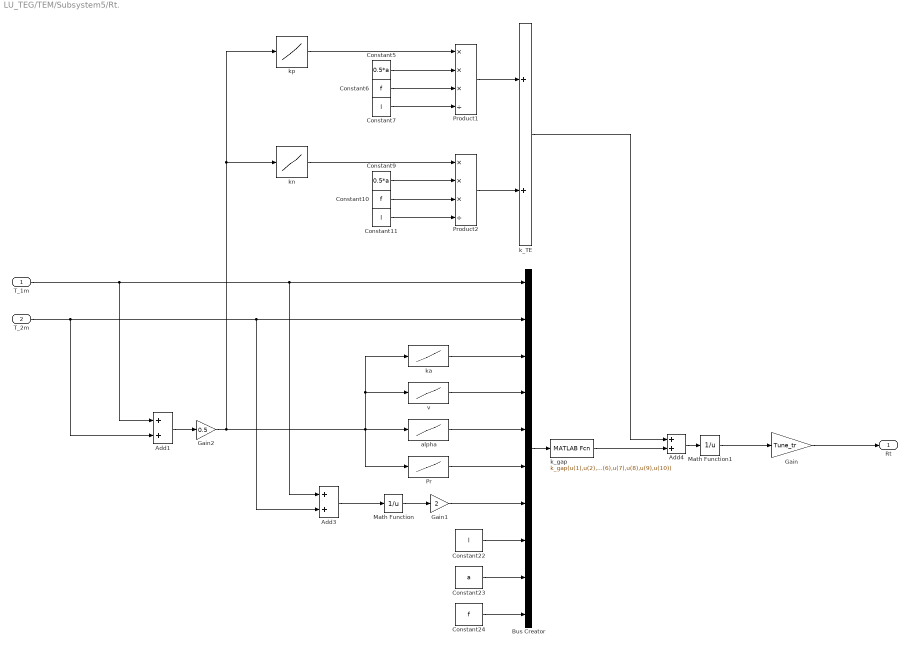
== system LU_TEG/TEM/Subsystem5/Rt. ==
  T_1m : Inport
  T_2m : Inport  Port=2
  Add1 : Sum
  Add3 : Sum
  Add4 : Sum
  Bus Creator : BusCreator  Inputs=10
  Constant10 : Constant  Value=f
  Constant11 : Constant  Value=l
  Constant22 : Constant  Value=l
  Constant23 : Constant  Value=a
  Constant24 : Constant  Value=f
  Constant5 : Constant  Value=0.5*a
  Constant6 : Constant  Value=f
  Constant7 : Constant  Value=l
  Constant9 : Constant  Value=0.5*a
  Gain : Gain  Gain=Tune_tr
  Gain1 : Gain  Gain=2
  Gain2 : Gain  Gain=0.5
  Math Function : Math  Operator=reciprocal  SaturateOnIntegerOverflow=on
  Math Function1 : Math  Operator=reciprocal  SaturateOnIntegerOverflow=on
  Pr : Lookup_n-D  NumberOfTableDimensions=1  BreakpointsForDimension1=|  Table=|  InterpMethod=Cubic spline  ExtrapMethod=Cubic spline  RndMeth=Simplest  InputSameDT=on
      BreakpointsForDimension1=|
      | [293
      | 313
      | 333
      | 353
      | 373
      | 393
      | 413
      | 433
      | 453
      | 473
      | 493
      | 513
      | 533
      | 553
      | 573
      | 593
      | 613
      | 633
      | 653
      | 673
      | 693
      | 713
      | 733
      | 753
      | 773
      | 793
      | 813
      | 833
      | 853
      | 873
      | 900
      | 920
      | 940
      | 960
      | 980
      | 1000
      | 1020
      | 1040
      | 1060
      | 1080
      | 1100
      | 1120
      | 1140
      | 1160
      | 1180
      | 1200
      | 1220
      | 1240
      | 1260
      | 1280
      | 1300
      | 1320
      | 1340
      | 1360
      | 1380
      | 1400
      | 1420
      | 1440
      | 1460
      | 1480]
      Table=|
      | [0.70868
      | 0.70388
      | 0.69972
      | 0.6964
      | 0.6924
      | 0.68912
      | 0.68696
      | 0.68536
      | 0.68376
      | 0.68216
      | 0.68056
      | 0.68
      | 0.68
      | 0.68
      | 0.68
      | 0.68
      | 0.68052
      | 0.68132
      | 0.68212
      | 0.68292
      | 0.68372
      | 0.68478
      | 0.68598
      | 0.68718
      | 0.68838
      | 0.68958
      | 0.69078
      | 0.69198
      | 0.69318
      | 0.69438
      | 0.696
      | 0.6972
      | 0.6984
      | 0.6996
      | 0.7008
      | 0.702
      | 0.7028
      | 0.7036
      | 0.7046
      | 0.7058
      | 0.707
      | 0.7078
      | 0.7086
      | 0.7094
      | 0.7102
      | 0.711
      | 0.7118
      | 0.7126
      | 0.7134
      | 0.7142
      | 0.715
      | 0.7158
      | 0.7166
      | 0.7174
      | 0.7182
      | 0.719
      | 0.7196
      | 0.7202
      | 0.7208
      | 0.7214
      | ]
  Product1 : Product  Inputs=***/
  Product2 : Product  Inputs=***/
  alpha : Lookup_n-D  NumberOfTableDimensions=1  BreakpointsForDimension1=|  Table=|  InterpMethod=Cubic spline  ExtrapMethod=Cubic spline  RndMeth=Simplest  InputSameDT=on
      BreakpointsForDimension1=|
      | [293
      | 313
      | 333
      | 353
      | 373
      | 393
      | 413
      | 433
      | 453
      | 473
      | 493
      | 513
      | 533
      | 553
      | 573
      | 593
      | 613
      | 633
      | 653
      | 673
      | 693
      | 713
      | 733
      | 753
      | 773
      | 793
      | 813
      | 833
      | 853
      | 873
      | 900
      | 920
      | 940
      | 960
      | 980
      | 1000
      | 1020
      | 1040
      | 1060
      | 1080
      | 1100
      | 1120
      | 1140
      | 1160
      | 1180
      | 1200
      | 1220
      | 1240
      | 1260
      | 1280
      | 1300
      | 1320
      | 1340
      | 1360
      | 1380
      | 1400
      | 1420
      | 1440
      | 1460
      | 1480]
      Table=|
      | [2.14551E-05
      | 2.42197E-05
      | 2.71451E-05
      | 3.01755E-05
      | 3.32992E-05
      | 3.65423E-05
      | 3.98418E-05
      | 4.32631E-05
      | 4.67259E-05
      | 5.03421E-05
      | 5.40342E-05
      | 5.77836E-05
      | 6.16602E-05
      | 6.5511E-05
      | 6.94474E-05
      | 7.35134E-05
      | 7.75786E-05
      | 8.18073E-05
      | 8.60163E-05
      | 9.03078E-05
      | 9.47366E-05
      | 9.91488E-05
      | 0.000103728
      | 0.000108175
      | 0.000112784
      | 0.000117529
      | 0.000122257
      | 0.000127153
      | 0.000132003
      | 0.000137003
      | 0.000142748
      | 0.000147552
      | 0.000152555
      | 0.00015755
      | 0.00016252
      | 0.000167688
      | 0.000172675
      | 0.000178002
      | 0.000183174
      | 0.000188489
      | 0.00019383
      | 0.000199144
      | 0.000204639
      | 0.000210134
      | 0.000215613
      | 0.000221274
      | 0.000226733
      | 0.000232362
      | 0.000238009
      | 0.000243871
      | 0.000249704
      | 0.000255298
      | 0.000261271
      | 0.000267061
      | 0.000273104
      | 0.00027932
      | 0.000285171
      | 0.000290933
      | 0.000297092
      | 0.000303417
      | ]
  k_TE : Sum
  k_gap : MATLABFcn  MATLABFcn=k_gap(u(1),u(2),u(3),u(4),u(5),u(6),u(7),u(8),u(9),u(10))
  ka : Lookup_n-D  NumberOfTableDimensions=1  BreakpointsForDimension1=|  Table=|  InterpMethod=Cubic spline  ExtrapMethod=Cubic spline  RndMeth=Simplest  InputSameDT=on
      BreakpointsForDimension1=|
      | [293
      | 313
      | 333
      | 353
      | 373
      | 393
      | 413
      | 433
      | 453
      | 473
      | 493
      | 513
      | 533
      | 553
      | 573
      | 593
      | 613
      | 633
      | 653
      | 673
      | 693
      | 713
      | 733
      | 753
      | 773
      | 793
      | 813
      | 833
      | 853
      | 873
      | 900
      | 920
      | 940
      | 960
      | 980
      | 1000
      | 1020
      | 1040
      | 1060
      | 1080
      | 1100
      | 1120
      | 1140
      | 1160
      | 1180
      | 1200
      | 1220
      | 1240
      | 1260
      | 1280
      | 1300
      | 1320
      | 1340
      | 1360
      | 1380
      | 1400
      | 1420
      | 1440
      | 1460
      | 1480]
      Table=|
      | [0.02568
      | 0.02716
      | 0.02861
      | 0.03003
      | 0.03142
      | 0.03279
      | 0.03412
      | 0.03544
      | 0.03673
      | 0.03801
      | 0.03926
      | 0.0405
      | 0.04172
      | 0.04293
      | 0.04413
      | 0.04531
      | 0.04648
      | 0.04764
      | 0.04879
      | 0.04993
      | 0.05106
      | 0.05218
      | 0.0533
      | 0.05441
      | 0.05551
      | 0.0566
      | 0.05769
      | 0.05877
      | 0.05985
      | 0.06092
      | 0.06276
      | 0.063736
      | 0.064712
      | 0.065668
      | 0.066604
      | 0.06754
      | 0.068464
      | 0.069388
      | 0.070298
      | 0.071194
      | 0.07209
      | 0.072962
      | 0.073834
      | 0.074696
      | 0.075548
      | 0.0764
      | 0.077236
      | 0.078072
      | 0.0789
      | 0.07972
      | 0.08054
      | 0.081336
      | 0.082132
      | 0.082924
      | 0.083712
      | 0.0845
      | 0.085262
      | 0.086024
      | 0.086786
      | 0.087548]
  kn : Lookup_n-D  NumberOfTableDimensions=1  BreakpointsForDimension1=N(:,1)  Table=N(:,4)  InterpMethod=Cubic spline  ExtrapMethod=Cubic spline  InternalRulePriority=Speed  RndMeth=Simplest  InputSameDT=on
  kp : Lookup_n-D  NumberOfTableDimensions=1  BreakpointsForDimension1=P(:,1)  Table=P(:,4)  InterpMethod=Cubic spline  ExtrapMethod=Cubic spline  InternalRulePriority=Speed  RndMeth=Simplest  InputSameDT=on
  v : Lookup_n-D  NumberOfTableDimensions=1  BreakpointsForDimension1=|  Table=|  InterpMethod=Cubic spline  ExtrapMethod=Cubic spline  RndMeth=Simplest  InputSameDT=on
      BreakpointsForDimension1=|
      | [293
      | 313
      | 333
      | 353
      | 373
      | 393
      | 413
      | 433
      | 453
      | 473
      | 493
      | 513
      | 533
      | 553
      | 573
      | 593
      | 613
      | 633
      | 653
      | 673
      | 693
      | 713
      | 733
      | 753
      | 773
      | 793
      | 813
      | 833
      | 853
      | 873
      | 900
      | 920
      | 940
      | 960
      | 980
      | 1000
      | 1020
      | 1040
      | 1060
      | 1080
      | 1100
      | 1120
      | 1140
      | 1160
      | 1180
      | 1200
      | 1220
      | 1240
      | 1260
      | 1280
      | 1300
      | 1320
      | 1340
      | 1360
      | 1380
      | 1400
      | 1420
      | 1440
      | 1460
      | 1480]
      Table=|
      | [1.50500000000000e-05
      | 1.69228000000000e-05
      | 1.88668000000000e-05
      | 2.08732000000000e-05
      | 2.29612000000000e-05
      | 2.51428000000000e-05
      | 2.74102000000000e-05
      | 2.97182000000000e-05
      | 3.20484000000000e-05
      | 3.45044000000000e-05
      | 3.69604000000000e-05
      | 3.95282000000000e-05
      | 4.21562000000000e-05
      | 4.48034000000000e-05
      | 4.75594000000000e-05
      | 5.03154000000000e-05
      | 5.31650000000000e-05
      | 5.60650000000000e-05
      | 5.89824000000000e-05
      | 6.19984000000000e-05
      | 6.50144000000000e-05
      | 6.81292000000000e-05
      | 7.12972000000000e-05
      | 7.44790000000000e-05
      | 7.77390000000000e-05
      | 8.09990000000000e-05
      | 8.43422000000000e-05
      | 8.77302000000000e-05
      | 9.11350000000000e-05
      | 9.46350000000000e-05
      | 9.93600000000000e-05
      | 0.000102936000000000
      | 0.000106512000000000
      | 0.000110160000000000
      | 0.000113880000000000
      | 0.000117600000000000
      | 0.000121440000000000
      | 0.000125280000000000
      | 0.000129160000000000
      | 0.000133080000000000
      | 0.000137000000000000
      | 0.000141000000000000
      | 0.000145000000000000
      | 0.000149060000000000
      | 0.000153180000000000
      | 0.000157300000000000
      | 0.000161460000000000
      | 0.000165620000000000
      | 0.000169860000000000
      | 0.000174180000000000
      | 0.000178500000000000
      | 0.000182860000000000
      | 0.000187220000000000
      | 0.000191640000000000
      | 0.000196120000000000
      | 0.000200600000000000
      | 0.000205200000000000
      | 0.000209800000000000
      | 0.000214400000000000
      | 0.000219000000000000]
  Rt : Outport
  wires:
  Gain/1 -> Rt/1
  Add3/1 -> Math Function/1
  T_1m/1 -> Add1/1, Bus Creator/1, Add3/1
  Bus Creator/1 -> k_gap/1
  k_gap/1 -> Add4/2
  Product1/1 -> k_TE/1
  Constant22/1 -> Bus Creator/8
  kp/1 -> Product1/1
  kn/1 -> Product2/1
  Constant5/1 -> Product1/2
  Constant6/1 -> Product1/3
  Product2/1 -> k_TE/2
  ka/1 -> Bus Creator/3
  Constant9/1 -> Product2/2
  alpha/1 -> Bus Creator/5
  Constant11/1 -> Product2/4
  v/1 -> Bus Creator/4
  Constant7/1 -> Product1/4
  Constant24/1 -> Bus Creator/10
  Pr/1 -> Bus Creator/6
  Constant23/1 -> Bus Creator/9
  Math Function/1 -> Gain1/1
  Constant10/1 -> Product2/3
  Gain1/1 -> Bus Creator/7
  Add4/1 -> Math Function1/1
  Math Function1/1 -> Gain/1
  Add1/1 -> Gain2/1
  Gain2/1 -> kp/1, kn/1, Pr/1, v/1, ka/1, alpha/1
  T_2m/1 -> Add1/2, Bus Creator/2, Add3/2
  k_TE/1 -> Add4/1

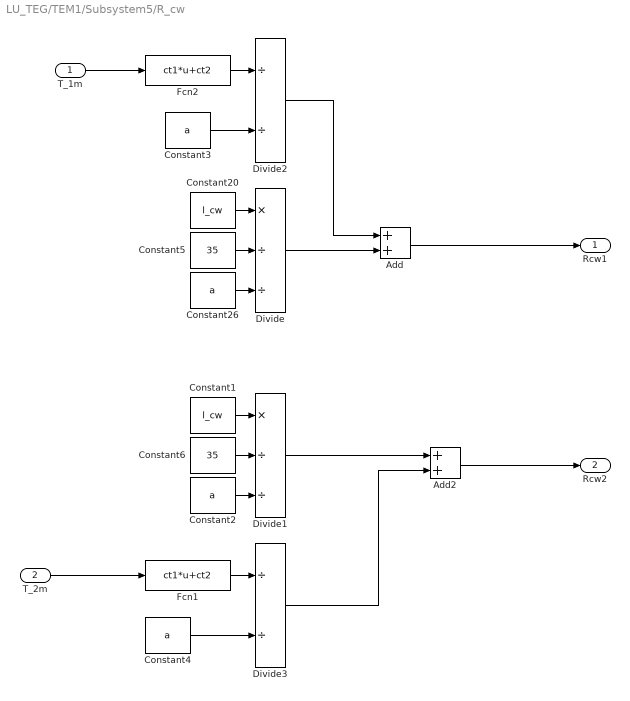
== system LU_TEG/TEM1/Subsystem5/R_cw ==
  T_1m : Inport
  T_2m : Inport  Port=2
  Add : Sum
  Add2 : Sum
  Constant1 : Constant  Value=l_cw
  Constant{2..4,26} (4 alike) : Constant  Value=a
  Constant20 : Constant  Value=l_cw
  Constant5 : Constant  Value=35
  Constant6 : Constant  Value=35
  Divide : Product  Inputs=*//
  Divide1 : Product  Inputs=*//
  Divide2 : Product  Inputs=//
  Divide3 : Product  Inputs=//
  Fcn1 : Fcn  Expr=ct1*u+ct2
  Fcn2 : Fcn  Expr=ct1*u+ct2
  Rcw1 : Outport
  Rcw2 : Outport  Port=2
  wires:
  Add2/1 -> Rcw2/1
  Divide3/1 -> Add2/2
  Constant4/1 -> Divide3/2
  Fcn1/1 -> Divide3/1
  Divide2/1 -> Add/1
  Constant3/1 -> Divide2/2
  Fcn2/1 -> Divide2/1
  Add/1 -> Rcw1/1
  Divide1/1 -> Add2/1
  Constant6/1 -> Divide1/2
  Constant2/1 -> Divide1/3
  Constant1/1 -> Divide1/1
  T_1m/1 -> Fcn2/1
  T_2m/1 -> Fcn1/1
  Divide/1 -> Add/2
  Constant5/1 -> Divide/2
  Constant26/1 -> Divide/3
  Constant20/1 -> Divide/1
